simulink model "testCollectorUnglazedCONF"  (R2016b)
settings: Solver=ode45  StartTime=0.0  StopTime=24*3600  MaxStep=1800  RelTol=1e-3  EnableMultiTasking=on
libraries: carnot x5
settings Model: Creator=drhf  LastModifiedBy=drhf
settings DataIOCC: LimitDataPoints=on  SaveFormat=Array
settings OptimizationCC: ExpressionDepthLimit=2147483647  LifeSpan=inf
settings DebuggingCC: UnderspecifiedInitializationDetection=Classic  MergeDetectMultiDrivingBlocksExec=none  SolverPrmCheckMsg=warning  StateNameClashWarn=warning  SFUnexpectedBacktrackingDiag=warning  SFNoUnconditionalDefaultTransitionDiag=warning  SFExecutionAtInitializationDiag=none
settings HardwareCC: ProdBitPerPointer=32  ProdBitPerSizeT=32  ProdBitPerPtrDiffT=32  ProdLargestAtomicFloat=None  ProdIntDivRoundTo=Undefined  ProdEndianess=Unspecified  ProdWordSize=32  ProdHWDeviceType=32-bit Generic
settings ModelReferenceCC: PropagateSignalLabelsOutOfModel=off
settings GRTTargetCC: TargetLangStandard=C89/C90 (ANSI)  GeneratePreprocessorConditionals=Disable all  CombineOutputUpdateFcns=off  GRTInterface=on
settings ConfigComp: CovMetricSettings=dw  CovHtmlReporting=on  CovSaveCumulativeToWorkspaceVar=on  CovSaveSingleToWorkspaceVar=on  CovExternalEMLEnable=off

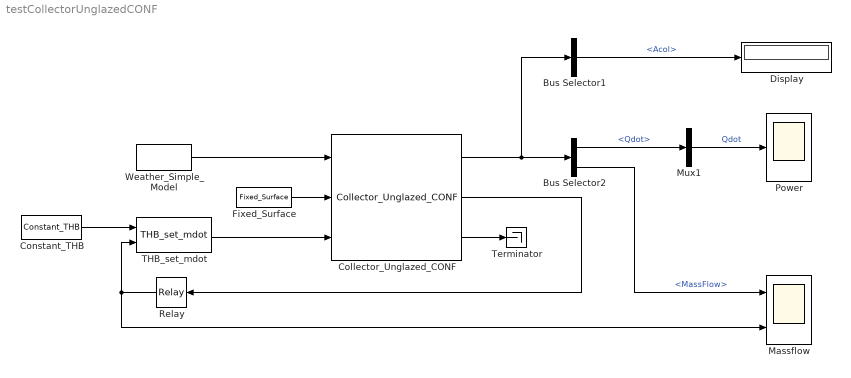
== system testCollectorUnglazedCONF ==
  Bus Selector1 : BusSelector  OutputSignals=Acol
  Bus Selector2 : BusSelector  OutputSignals=Qdot,THBout.MassFlow
  Collector_Unglazed_CONF : carnot/Source/Solar_Thermal/Collector_Unglazed_CONF  tini=22  Ncollector=1  PathName='C:\repos\carnot_svn\trunk\internal\library_simulink\Source\Solar_Thermal\Collector_Unglazed_CONF\parameter_set\'  FileName='USTC_set1.mat'  userPath=off  userParam=off  acol=5  len=2.3  nodes=5  fta=0.75  eps=0.9  u0l=4  u0c=10  u0g=4  u1l=3  u1c=3  u1g=1.5  u1e=0.01  hi=100  capa=7000  capf=2000  SensorTimeConstant=10  dplin=10  dpqua=10
  Constant_THB : carnot/Source/Simple/Constant_THB  t=40  mdot=100/3600  p=1e5  mID=No Pressure Drop  fluid=Water  mix=0  mix2=0  mix3=0  dia=0.02  hgt=0
  Display : Display
  Fixed_Surface : carnot/Weather/Fixed_Surface  colangle=30  colazi=0  colrot=0
  Massflow : Scope  NumInputPorts=2
  Mux1 : Mux  Inputs=1
  Power : Scope
  Relay : Relay  OnSwitchValue=47  OffSwitchValue=42  OnOutputValue=100/3600
  THB_set_mdot : carnot/Source/Simple/THB_set_mdot
  Terminator : Terminator
  Weather_Simple_Model : carnot/Weather/Weather_Simple_Model  lat=60  Ibn=900  Idg=100  tamb=5  deltaTsky=-6  rh=50  precip="10e-3/24/3600           % 10 mm in 24 h"  cloud=0.125  p=1013e2  vw=1  wdir=270
  wires:
  Constant_THB/1 -> THB_set_mdot/1
  THB_set_mdot/1 -> Collector_Unglazed_CONF/3
  Fixed_Surface/1 -> Collector_Unglazed_CONF/2
  Weather_Simple_Model/1 -> Collector_Unglazed_CONF/1
  Relay/1 -> Massflow/2, THB_set_mdot/2
  Collector_Unglazed_CONF/2 -> Relay/1
  Bus Selector2/1 -> Mux1/1  "<Qdot>"
  Collector_Unglazed_CONF/3 -> Terminator/1
  Mux1/1 -> Power/1  "Qdot"
  Collector_Unglazed_CONF/1 -> Bus Selector1/1, Bus Selector2/1
  Bus Selector2/2 -> Massflow/1  "<MassFlow>"
  Bus Selector1/1 -> Display/1  "<Acol>"
